simulink model "PCS_Model"  (R2019b)
settings: Solver=VariableStepAuto  StartTime=0.0  StopTime=10.0  RelTol=1e-3
undefined symbols (not defined in the file): P1, T1, V1
libraries: simulink x1
settings Model: Creator=keatonnichols  LastModifiedBy=keatonnichols

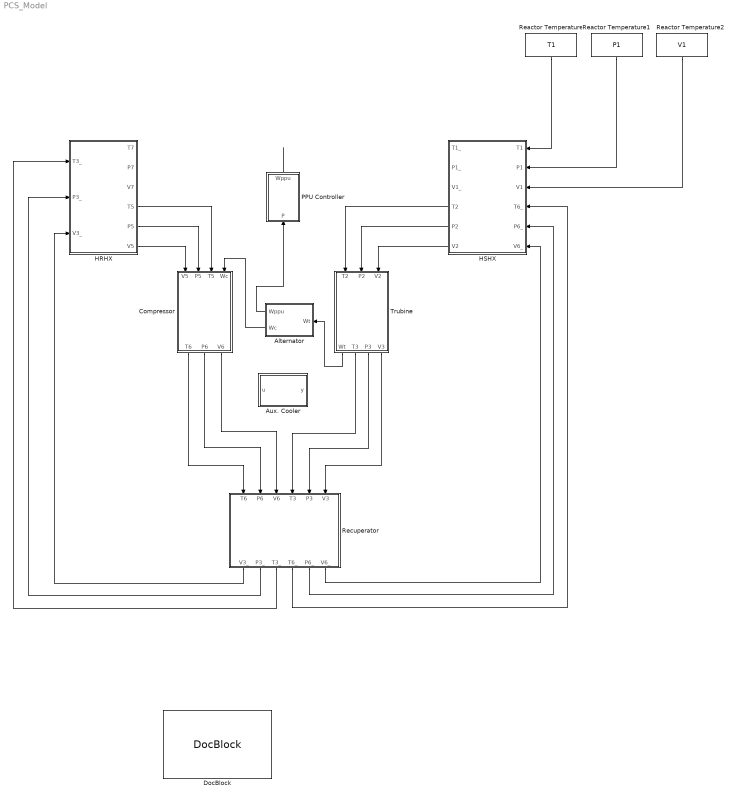
== system PCS_Model ==
  Alternator : MATLAB Function  TreatAsAtomicUnit=on
  Aux. Cooler : MATLAB Function  TreatAsAtomicUnit=on
  Compressor : MATLAB Function  TreatAsAtomicUnit=on
  DocBlock : simulink/Model-Wide Utilities/DocBlock  Tag=|  Description=|  DocumentType=Text
      Tag=|
      | HSHX : 1 (8) --> 2
      | Turbine : 2 --> 3
      | Recuperator : 3 (7) --> 4 (8)
      | HRHX : 4 --> 5 (6)
      | Compressor : 5 --> 7
      Description=|
      | HSHX : 1 (8) --> 2
      | Turbine : 2 --> 3
      | Recuperator : 3 (7) --> 4 (8)
      | HRHX : 4 --> 5 (6)
      | Compressor : 5 --> 7
      content=|
      | HSHX : 6' --> 2
      | Turbine : 2 --> 3
      | Recuperator : 3 + 6 --> 3' + 6'
      | HRHX : 3' --> 5
      | Compressor : 5 --> 6
  HRHX : MATLAB Function  TreatAsAtomicUnit=on
  HSHX : MATLAB Function  TreatAsAtomicUnit=on
  PPU Controller : MATLAB Function  TreatAsAtomicUnit=on
  Reactor Temperature : Constant  Value=T1
  Reactor Temperature1 : Constant  Value=P1
  Reactor Temperature2 : Constant  Value=V1
  Recuperator : MATLAB Function  TreatAsAtomicUnit=on
  Trubine : MATLAB Function  TreatAsAtomicUnit=on
  wires:
  HSHX/6(V2) -> Trubine/3(V2)
  HSHX/5(P2) -> Trubine/2(P2)
  HSHX/4(T2) -> Trubine/1(T2)
  Trubine/2(T3) -> Recuperator/4(T3)
  Trubine/3(P3) -> Recuperator/5(P3)
  Trubine/4(V3) -> Recuperator/6(V3)
  Compressor/3(V6) -> Recuperator/3(V6)
  Compressor/2(P6) -> Recuperator/2(P6)
  Compressor/1(T6) -> Recuperator/1(T6)
  Recuperator/3(T3_) -> HRHX/1(T3_)
  Recuperator/2(P3_) -> HRHX/2(P3_)
  Recuperator/1(V3_) -> HRHX/3(V3_)
  Recuperator/4(T6_) -> HSHX/4(T6_)
  Recuperator/5(P6_) -> HSHX/5(P6_)
  Recuperator/6(V6_) -> HSHX/6(V6_)
  HRHX/6(V5) -> Compressor/1(V5)
  HRHX/5(P5) -> Compressor/2(P5)
  HRHX/4(T5) -> Compressor/3(T5)
  Trubine/1(Wt) -> Alternator/1(Wt)
  Alternator/2(Wc) -> Compressor/4(Wc)
  Alternator/1(Wppu) -> PPU Controller/1(P)
  Reactor Temperature/1 -> HSHX/1(T1)
  Reactor Temperature1/1 -> HSHX/2(P1)
  Reactor Temperature2/1 -> HSHX/3(V1)
  PPU Controller/1(Wppu) -> ?

== matlab function PCS_Model/Compressor ==
  data: V5 input; P5 input; T5 input; T6 output; P6 output; V6 output; Wc input
function [T6,P6,V6] = fcn(V5,P5,T5,Wc)

;

== matlab function PCS_Model/Trubine ==
  data: Wt output; T2 input; T3 output; P2 input; V2 input; P3 output; V3 output
function [Wt,T3,P3,V3] = fcn(T2,P2,V2)
%HeXe Properties

R = 558; %J/kg-K
rho = 14.229; %kg/m^3

;

== matlab function PCS_Model/Alternator ==
  data: Wppu output; Wt input; Wc output
function [Wppu,Wc] = fcn(Wt)

;

== matlab function PCS_Model/Aux. Cooler ==
  data: u input; y output
function y = fcn(u)

y = u;

== matlab function PCS_Model/Recuperator ==
  data: V3_ output; P3_ output; T3_ output; T6 input; T6_ output; P6 input; V6 input; T3 input; P3 input; V3 input; P6_ output; V6_ output
function [V3_,P3_,T3_,T6_,P6_,V6_] = fcn(T6,P6,V6,T3,P3,V3)

;

== matlab function PCS_Model/HRHX ==
  data: T7 output; P7 output; V7 output; T3_ input; T5 output; P3_ input; V3_ input; P5 output; V5 output
function [T7,P7,V7,T5,P5,V5] = fcn(T3_,P3_,V3_)

;

== matlab function PCS_Model/HSHX ==
  data: T1_ output; P1_ output; V1_ output; T1 input; P1 input; V1 input; T2 output; T6_ input; P6_ input; V6_ input; P2 output; V2 output
function [T1_,P1_,V1_,T2,P2,V2] = fcn(T1,P1,V1,T6_,P6_,V6_)

%T1 is temperature of flow coming from reactor


;

== matlab function PCS_Model/PPU Controller ==
  data: P input; Wppu output
function Wppu = fcn(P)

;
